simulink model "rxPacketGenerator"  (R2022a)
settings: Solver=FixedStepDiscrete  StartTime=0.0  StopTime=simTime  RelTol=1e-3
model workspace (MAT data in the model file):
  Sig = Simulink.Signal
  Sig.DataType = 'auto'
  Sig.Dimensions = -1
  Sig.DimensionsMode = 'auto'
  Sig.Complexity = 'auto'
  Sig.SampleTime = -1
  Sig.SamplingMode = 'auto'
libraries: dspsrcs4 x14
settings Model: DataTypeOverride=Off  Creator=ASAHIN  LastModifiedBy=alpha
settings SolverCC: AlgebraicLoopSolver=TrustRegion
settings OptimizationCC: BlockReduction=off  ConditionallyExecuteInputs=off  DefaultParameterBehavior=Inlined  InheritOutputTypeSmallerThanSingle=on
settings DebuggingCC: AlgebraicLoopMsg=error  SingleTaskRateTransMsg=error  UnconnectedInputMsg=warning  UnconnectedOutputMsg=warning  UnconnectedLineMsg=warning  SFMachineParentedDataDiag=warning
settings HardwareCC: ProdBitPerPointer=32  ProdBitPerSizeT=32  ProdBitPerPtrDiffT=32  ProdLargestAtomicFloat=None  ProdIntDivRoundTo=Undefined  ProdEndianess=Unspecified  ProdWordSize=32  ProdHWDeviceType=ASIC/FPGA->ASIC/FPGA  TargetBitPerPointer=64  TargetBitPerSizeT=64  TargetBitPerPtrDiffT=64  TargetLongLongMode=on  TargetIntDivRoundTo=Zero  TargetEndianess=LittleEndian  TargetWordSize=64  TargetHWDeviceType=Custom Processor->MATLAB Host Computer  ProdEqTarget=off
settings RTWCC: DLArmComputeVersion=19.05

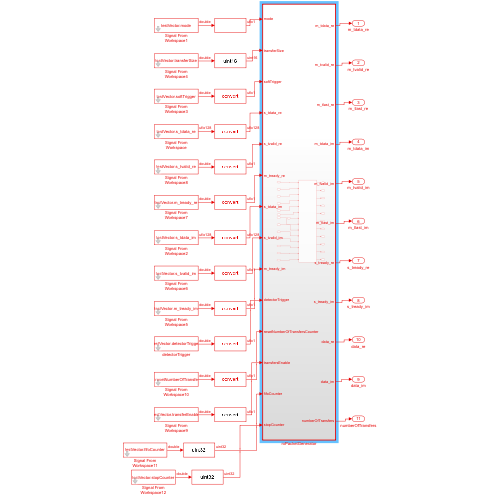
[thumbnail: Simulink's stored preview of the top-level diagram]
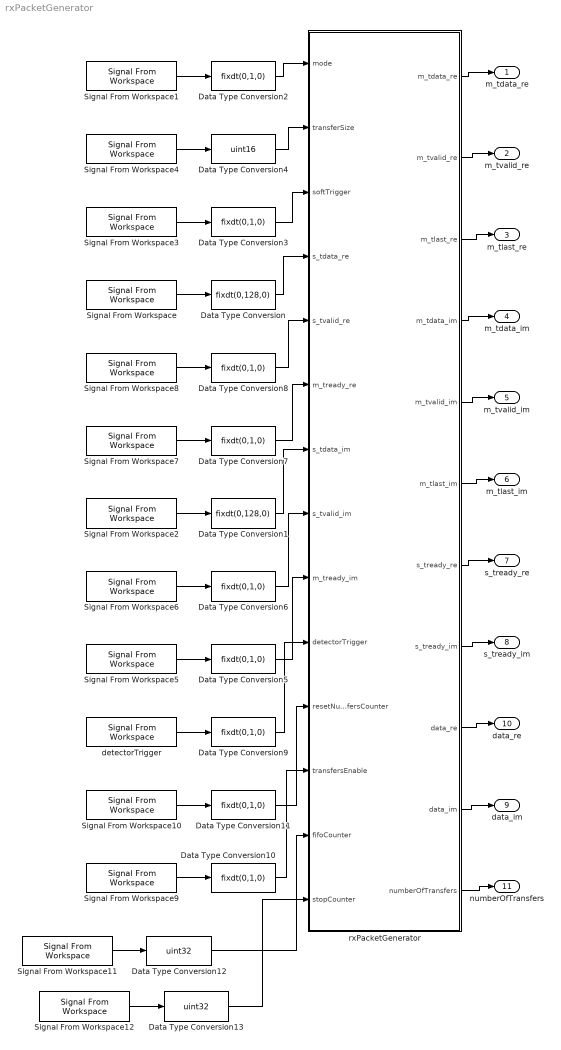
== system rxPacketGenerator ==
  Data Type Conversion : DataTypeConversion  OutDataTypeStr=fixdt(0,128,0)  SaturateOnIntegerOverflow=off  RndMeth=Floor
  Data Type Conversion1 : DataTypeConversion  OutDataTypeStr=fixdt(0,128,0)  SaturateOnIntegerOverflow=off  RndMeth=Floor
  Data Type Conversion{2..3,5..11} (9 alike) : DataTypeConversion  OutDataTypeStr=fixdt(0,1,0)  SaturateOnIntegerOverflow=off  RndMeth=Floor
  Data Type Conversion12 : DataTypeConversion  OutDataTypeStr=uint32  SaturateOnIntegerOverflow=off  RndMeth=Floor
  Data Type Conversion13 : DataTypeConversion  OutDataTypeStr=uint32  SaturateOnIntegerOverflow=off  RndMeth=Floor
  Data Type Conversion4 : DataTypeConversion  OutDataTypeStr=uint16  SaturateOnIntegerOverflow=off  RndMeth=Floor
  Signal From Workspace : dspsrcs4/Signal From Workspace  X=testVector.s_tdata_re  Ts=1  nsamps=1  OutputAfterFinalValue=Setting to zero  ignoreOrWarnInputAndFrameLengths=off  OutputFrames=off
  Signal From Workspace1 : dspsrcs4/Signal From Workspace  X=testVector.mode  Ts=1  nsamps=1  OutputAfterFinalValue=Setting to zero  ignoreOrWarnInputAndFrameLengths=off  OutputFrames=off
  Signal From Workspace10 : dspsrcs4/Signal From Workspace  X=testVector.resetNumberOfTransfersCounter  Ts=1  nsamps=1  OutputAfterFinalValue=Setting to zero  ignoreOrWarnInputAndFrameLengths=off  OutputFrames=off
  Signal From Workspace11 : dspsrcs4/Signal From Workspace  X=testVector.fifoCounter  Ts=1  nsamps=1  OutputAfterFinalValue=Setting to zero  ignoreOrWarnInputAndFrameLengths=off  OutputFrames=off
  Signal From Workspace12 : dspsrcs4/Signal From Workspace  X=testVector.stopCounter  Ts=1  nsamps=1  OutputAfterFinalValue=Setting to zero  ignoreOrWarnInputAndFrameLengths=off  OutputFrames=off
  Signal From Workspace2 : dspsrcs4/Signal From Workspace  X=testVector.s_tdata_im  Ts=1  nsamps=1  OutputAfterFinalValue=Setting to zero  ignoreOrWarnInputAndFrameLengths=off  OutputFrames=off
  Signal From Workspace3 : dspsrcs4/Signal From Workspace  X=testVector.softTrigger  Ts=1  nsamps=1  OutputAfterFinalValue=Setting to zero  ignoreOrWarnInputAndFrameLengths=off  OutputFrames=off
  Signal From Workspace4 : dspsrcs4/Signal From Workspace  X=testVector.transferSize  Ts=1  nsamps=1  OutputAfterFinalValue=Setting to zero  ignoreOrWarnInputAndFrameLengths=off  OutputFrames=off
  Signal From Workspace5 : dspsrcs4/Signal From Workspace  X=testVector.m_tready_im  Ts=1  nsamps=1  OutputAfterFinalValue=Setting to zero  ignoreOrWarnInputAndFrameLengths=off  OutputFrames=off
  Signal From Workspace6 : dspsrcs4/Signal From Workspace  X=testVector.s_tvalid_im  Ts=1  nsamps=1  OutputAfterFinalValue=Setting to zero  ignoreOrWarnInputAndFrameLengths=off  OutputFrames=off
  Signal From Workspace7 : dspsrcs4/Signal From Workspace  X=testVector.m_tready_re  Ts=1  nsamps=1  OutputAfterFinalValue=Setting to zero  ignoreOrWarnInputAndFrameLengths=off  OutputFrames=off
  Signal From Workspace8 : dspsrcs4/Signal From Workspace  X=testVector.s_tvalid_re  Ts=1  nsamps=1  OutputAfterFinalValue=Setting to zero  ignoreOrWarnInputAndFrameLengths=off  OutputFrames=off
  Signal From Workspace9 : dspsrcs4/Signal From Workspace  X=testVector.transferEnable  Ts=1  nsamps=1  OutputAfterFinalValue=Setting to zero  ignoreOrWarnInputAndFrameLengths=off  OutputFrames=off
  detectorTrigger : dspsrcs4/Signal From Workspace  X=testVector.detectorTrigger  Ts=1  nsamps=1  OutputAfterFinalValue=Setting to zero  ignoreOrWarnInputAndFrameLengths=off  OutputFrames=off
  rxPacketGenerator : Subsystem  TreatAsAtomicUnit=on
  m_tdata_re : Outport
  m_tvalid_re : Outport  Port=2
  m_tlast_re : Outport  Port=3
  m_tdata_im : Outport  Port=4
  m_tvalid_im : Outport  Port=5
  m_tlast_im : Outport  Port=6
  s_tready_re : Outport  Port=7
  s_tready_im : Outport  Port=8
  data_im : Outport  Port=9
  data_re : Outport  Port=10
  numberOfTransfers : Outport  Port=11
  wires:
  Data Type Conversion5/1 -> rxPacketGenerator/9(m_tready_im)
  Data Type Conversion8/1 -> rxPacketGenerator/5(s_tvalid_re)
  Data Type Conversion2/1 -> rxPacketGenerator/1(mode)
  Data Type Conversion4/1 -> rxPacketGenerator/2(transferSize)
  Data Type Conversion7/1 -> rxPacketGenerator/6(m_tready_re)
  Data Type Conversion10/1 -> rxPacketGenerator/12(transfersEnable)
  Data Type Conversion6/1 -> rxPacketGenerator/8(s_tvalid_im)
  rxPacketGenerator/1(m_tdata_re) -> m_tdata_re/1
  Signal From Workspace2/1 -> Data Type Conversion1/1
  rxPacketGenerator/5(m_tvalid_im) -> m_tvalid_im/1
  rxPacketGenerator/4(m_tdata_im) -> m_tdata_im/1
  rxPacketGenerator/8(s_tready_im) -> s_tready_im/1
  rxPacketGenerator/9(data_re) -> data_re/1
  Signal From Workspace8/1 -> Data Type Conversion8/1
  rxPacketGenerator/11(numberOfTransfers) -> numberOfTransfers/1
  rxPacketGenerator/10(data_im) -> data_im/1
  rxPacketGenerator/3(m_tlast_re) -> m_tlast_re/1
  rxPacketGenerator/2(m_tvalid_re) -> m_tvalid_re/1
  Signal From Workspace3/1 -> Data Type Conversion3/1
  Data Type Conversion9/1 -> rxPacketGenerator/10(detectorTrigger)
  Data Type Conversion3/1 -> rxPacketGenerator/3(softTrigger)
  Data Type Conversion/1 -> rxPacketGenerator/4(s_tdata_re)
  Signal From Workspace1/1 -> Data Type Conversion2/1
  Data Type Conversion1/1 -> rxPacketGenerator/7(s_tdata_im)
  detectorTrigger/1 -> Data Type Conversion9/1
  Signal From Workspace6/1 -> Data Type Conversion6/1
  Signal From Workspace7/1 -> Data Type Conversion7/1
  rxPacketGenerator/7(s_tready_re) -> s_tready_re/1
  rxPacketGenerator/6(m_tlast_im) -> m_tlast_im/1
  Signal From Workspace5/1 -> Data Type Conversion5/1
  Signal From Workspace/1 -> Data Type Conversion/1
  Data Type Conversion11/1 -> rxPacketGenerator/11(resetNumberOfTransfersCounter)
  Signal From Workspace4/1 -> Data Type Conversion4/1
  Signal From Workspace10/1 -> Data Type Conversion11/1
  Signal From Workspace9/1 -> Data Type Conversion10/1
  Data Type Conversion12/1 -> rxPacketGenerator/13(fifoCounter)
  Signal From Workspace11/1 -> Data Type Conversion12/1
  Data Type Conversion13/1 -> rxPacketGenerator/14(stopCounter)
  Signal From Workspace12/1 -> Data Type Conversion13/1

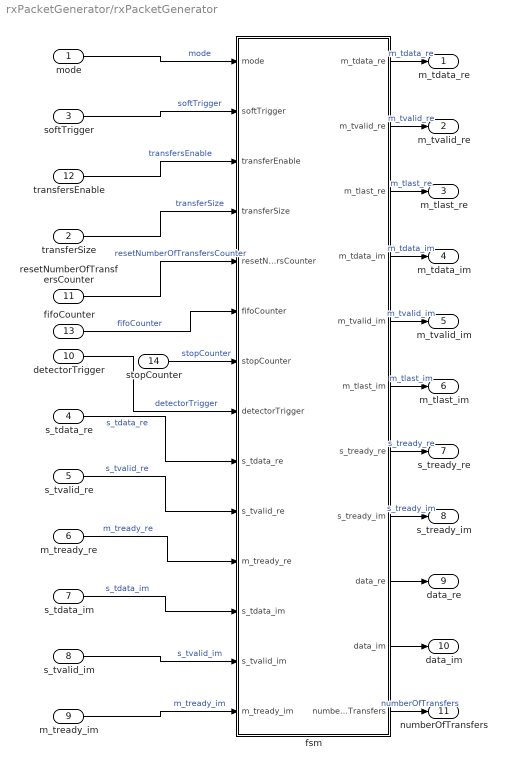
== system rxPacketGenerator/rxPacketGenerator ==
  mode : Inport
  transferSize : Inport  Port=2
  softTrigger : Inport  Port=3
  s_tdata_re : Inport  Port=4
  s_tvalid_re : Inport  Port=5
  m_tready_re : Inport  Port=6
  s_tdata_im : Inport  Port=7
  s_tvalid_im : Inport  Port=8
  m_tready_im : Inport  Port=9
  detectorTrigger : Inport  Port=10
  resetNumberOfTransfersCounter : Inport  Port=11
  transfersEnable : Inport  Port=12
  fifoCounter : Inport  Port=13
  stopCounter : Inport  Port=14
  fsm : MATLAB Function  TreatAsAtomicUnit=on
  m_tdata_re : Outport
  m_tvalid_re : Outport  Port=2
  m_tlast_re : Outport  Port=3
  m_tdata_im : Outport  Port=4
  m_tvalid_im : Outport  Port=5
  m_tlast_im : Outport  Port=6
  s_tready_re : Outport  Port=7
  s_tready_im : Outport  Port=8
  data_re : Outport  Port=9
  data_im : Outport  Port=10
  numberOfTransfers : Outport  Port=11
  wires:
  transferSize/1 -> fsm/4(transferSize)  "transferSize"
  s_tdata_re/1 -> fsm/9(s_tdata_re)  "s_tdata_re"
  m_tready_im/1 -> fsm/14(m_tready_im)  "m_tready_im"
  s_tvalid_re/1 -> fsm/10(s_tvalid_re)  "s_tvalid_re"
  fsm/11(numberOfTransfers) -> numberOfTransfers/1  "numberOfTransfers"
  fsm/3(m_tlast_re) -> m_tlast_re/1  "m_tlast_re"
  fsm/8(s_tready_im) -> s_tready_im/1  "s_tready_im"
  fsm/9(data_re) -> data_re/1
  fsm/10(data_im) -> data_im/1
  fsm/5(m_tvalid_im) -> m_tvalid_im/1  "m_tvalid_im"
  fsm/6(m_tlast_im) -> m_tlast_im/1  "m_tlast_im"
  fsm/4(m_tdata_im) -> m_tdata_im/1  "m_tdata_im"
  fsm/7(s_tready_re) -> s_tready_re/1  "s_tready_re"
  softTrigger/1 -> fsm/2(softTrigger)  "softTrigger"
  s_tvalid_im/1 -> fsm/13(s_tvalid_im)  "s_tvalid_im"
  m_tready_re/1 -> fsm/11(m_tready_re)  "m_tready_re"
  fsm/2(m_tvalid_re) -> m_tvalid_re/1  "m_tvalid_re"
  fsm/1(m_tdata_re) -> m_tdata_re/1  "m_tdata_re"
  detectorTrigger/1 -> fsm/8(detectorTrigger)  "detectorTrigger"
  s_tdata_im/1 -> fsm/12(s_tdata_im)  "s_tdata_im"
  mode/1 -> fsm/1(mode)  "mode"
  transfersEnable/1 -> fsm/3(transferEnable)  "transfersEnable"
  resetNumberOfTransfersCounter/1 -> fsm/5(resetNumberOfTransfersCounter)  "resetNumberOfTransfersCounter"
  fifoCounter/1 -> fsm/6(fifoCounter)  "fifoCounter"
  stopCounter/1 -> fsm/7(stopCounter)  "stopCounter"

== matlab function rxPacketGenerator/fsm ==
  settings: fimath=fimath('RoundingMethod', 'Floor','OverflowAction', 'Wrap','ProductMode', 'FullPrecision', 'SumMode', 'FullPrecision')
  data: mode input; softTrigger input; transferEnable input; transferSize input; resetNumberOfTransfersCounter input; fifoCounter input; stopCounter input; m_tdata_re output; detectorTrigger input; s_tdata_re input; s_tvalid_re input; m_tready_re input; s_tdata_im input; s_tvalid_im input; m_tready_im input; m_tvalid_re output; m_tlast_re output; m_tdata_im output; m_tvalid_im output; m_tlast_im output; s_tready_re output; s_tready_im output; data_re output; data_im output; numberOfTransfers output
function [m_tdata_re, m_tvalid_re, m_tlast_re,m_tdata_im, m_tvalid_im, m_tlast_im, s_tready_re, s_tready_im, data_re, data_im, numberOfTransfers]   = fcn_stateMachine(mode,...
                                                                                    softTrigger, transferEnable,  transferSize, resetNumberOfTransfersCounter, fifoCounter,stopCounter,...
                                                                                    detectorTrigger, ...
                                                                                    s_tdata_re, s_tvalid_re, m_tready_re, ...
                                                                                    s_tdata_im, s_tvalid_im, m_tready_im)
    %% Initialize Registers
    persistent counter_numberOfTransfers_reg;
    if isempty(counter_numberOfTransfers_reg)
        counter_numberOfTransfers_reg = uint32(0);
    end
 
    
    persistent counter_reg;
    if isempty(counter_reg)
        counter_reg = uint16(0);
    end
    
    persistent counterCompleted_reg;
    if isempty(counterCompleted_reg)
        counterCompleted_reg = fi(0,0,1,0);
    end


    persistent state_reg;
    if isempty(state_reg)
        state_reg = fi(0,0,1,0);
    end    

    
    persistent softTrigger_reg;
    if isempty(softTrigger_reg)
        softTrigger_reg = fi(0,0,1,0);
    end

    persistent isThereEnoughRoom_reg;
    if isempty(isThereEnoughRoom_reg)
        isThereEnoughRoom_reg = false;
    end    
    
    %% Set outputs (delayed)
    m_tdata_re = s_tdata_re;
    data_re = s_tdata_re;
    
    m_tvalid_re = state_reg == fi(1,0,1,0) && s_tvalid_re == fi(1,0,1,0) && s_tvalid_im == fi(1,0,1,0);
    s_tready_re = state_reg == fi(1,0,1,0) && m_tready_re == fi(1,0,1,0) && m_tready_im == fi(1,0,1,0);   

    m_tdata_im = s_tdata_im;
    data_im = s_tdata_im;
    
    m_tvalid_im = state_reg == fi(1,0,1,0) && s_tvalid_im == fi(1,0,1,0) && s_tvalid_im == fi(1,0,1,0);
    s_tready_im = state_reg == fi(1,0,1,0) && m_tready_im == fi(1,0,1,0) && m_tready_im == fi(1,0,1,0);   


    softTrigger_risingEdge = softTrigger_reg == fi(0,0,1,0) && softTrigger == fi(1,0,1,0);
    
    if mode == fi(0,0,1,0)
        trigger = softTrigger_risingEdge;
    else
        trigger = softTrigger_risingEdge || detectorTrigger;
    end

    numberOfTransfers = counter_numberOfTransfers_reg;

    
    
    
    %% Update Registers
    switch state_reg
        case fi(0,0,1,0) % wait
            changeState = trigger == fi(1,0,1,0) && transferEnable == fi(1,0,1,0) && transferSize>0 && isThereEnoughRoom_reg == true;
            if changeState == fi(1,0,1,0)
                state_reg = fi(1,0,1,0);
            end
            counter_reg = transferSize;
            if resetNumberOfTransfersCounter == fi(1,0,1,0)
                counter_numberOfTransfers_reg = uint32(0);
            end
            counterCompleted_reg = fi(0,0,1,0);
        case fi(1,0,1,0) % count
            if s_tvalid_re == fi(1,0,1,0) && m_tready_re == fi(1,0,1,0) && s_tvalid_im == fi(1,0,1,0) && m_tready_im == fi(1,0,1,0)
                if counter_reg == 1
                    state_reg = fi(0,0,1,0);
                    counterCompleted_reg = fi(1,0,1,0);
                    counter_numberOfTransfers_reg = counter_numberOfTransfers_reg + 1;
                end
                counter_reg = counter_reg - 1;
            end
    end         
    softTrigger_reg = softTrigger;
    isThereEnoughRoom_reg = fifoCounter<stopCounter;

    %% Set outputs (not delayed)
    m_tlast_re = counterCompleted_reg == 1;
    m_tlast_im = counterCompleted_reg == 1;
